simulink model "torque_control_180"  (R2021a)
settings: Solver=FixedStepAuto  StartTime=0.0  StopTime=1  FixedStep=1e-6  MaxStep=1e-6  RelTol=1e-3
values from neighbouring files (symbols this model uses):
  P = 8    [Arrow_86EMB3S98F_specs.m]    (also in M_2311P_specs.m)
undefined symbols (not defined in the file or in its folder): DiscIntNeverNeededParam, J, k1, k2, lambda_md, lls, rs, vdc
libraries: simulink x19, spsIGBTDiodeLib x6, spsSeriesRLCBranchLib x4, spsVoltageMeasurementLib x4, spsControlledCurrentSourceLib x3, spsGroundLib x2, spsControlledVoltageSourceLib x1, spspowerguiLib x1
settings Model: Creator=zlfen019.stu  LastModifiedBy=zlfen019.stu
settings DataIOCC: ReturnWorkspaceOutputs=off

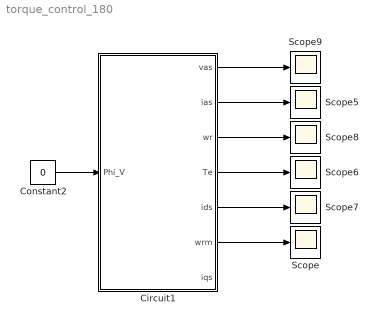
== system torque_control_180 ==
  Circuit1 : Subsystem
  Constant2 : Constant  Value=0
  Scope{,5..9} (6 alike) : Scope
  wires:
  Constant2/1 -> Circuit1/1(Phi_V)
  Circuit1/4(Te) -> Scope6/1
  Circuit1/5(ids) -> Scope7/1
  Circuit1/3(wr) -> Scope8/1
  Circuit1/2(ias) -> Scope5/1
  Circuit1/1(vas) -> Scope9/1
  Circuit1/6(wrm) -> Scope/1

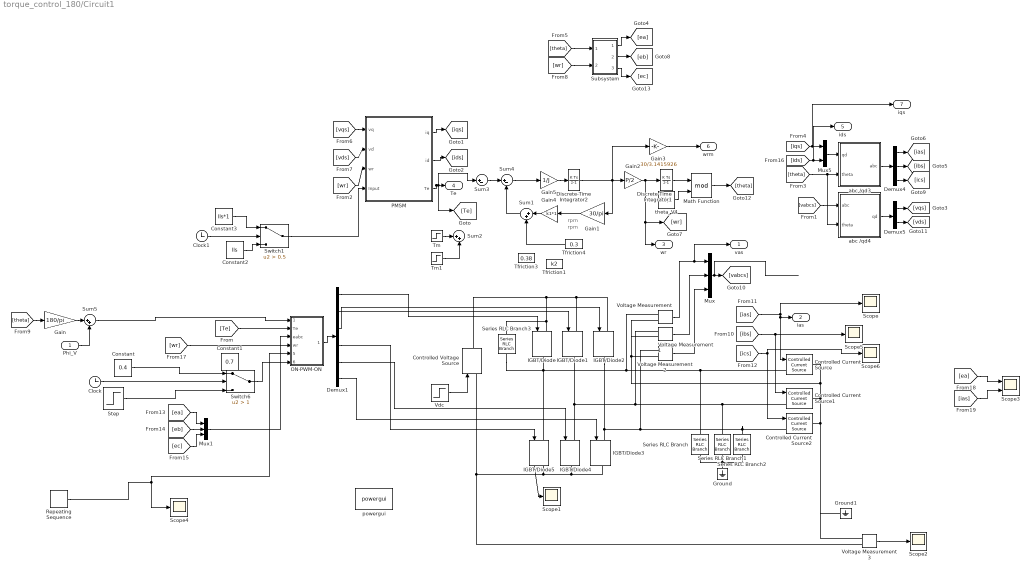
== system torque_control_180/Circuit1 ==
  note: rpm
  note: rpm
  Phi_V : Inport
  Clock : Clock
  Clock1 : Clock
  Constant : Constant  Value=0.4
  Constant1 : Constant  Value=0.7
  Constant2 : Constant  Value=lls
  Constant3 : Constant  Value=lls*1
  Controlled Current Source : spsControlledCurrentSourceLib/Controlled Current Source  Initialize=on  Source_Type=AC  Amplitude=0  Phase=0  Frequency=0  Measurements=None
  Controlled Current Source1 : spsControlledCurrentSourceLib/Controlled Current Source  Initialize=on  Source_Type=AC  Amplitude=0  Phase=0  Frequency=0  Measurements=None
  Controlled Current Source2 : spsControlledCurrentSourceLib/Controlled Current Source  Initialize=on  Source_Type=AC  Amplitude=0  Phase=0  Frequency=0  Measurements=None
  Controlled Voltage Source : spsControlledVoltageSourceLib/Controlled Voltage Source  Initialize=off  Source_Type=AC  Amplitude=0  Phase=0  Frequency=0  Measurements=None
  Demux1 : Demux  Outputs=6
  Demux4 : Demux  Outputs=3
  Demux5 : Demux  Outputs=2
  Discrete-Time Integrator1 : DiscreteIntegrator  SampleTime=-1  ICPrevOutput=DiscIntNeverNeededParam  ICPrevScaledInput=DiscIntNeverNeededParam
  Discrete-Time Integrator2 : DiscreteIntegrator  SampleTime=-1  ICPrevOutput=DiscIntNeverNeededParam  ICPrevScaledInput=DiscIntNeverNeededParam
  Gain : Gain  Gain=180/pi
  Gain1 : Gain  Gain=30/pi
  Gain2 : Gain  Gain=P/2
  Gain3 : Gain  Gain=30/3.1415926
  Gain4 : Gain  Gain=k1*1
  Gain5 : Gain  Gain=1/J
  Ground : spsGroundLib/Ground  LConnTagsString=a
  Ground1 : spsGroundLib/Ground  LConnTagsString=a
  IGBT/Diode{,1..4} (5 alike) : spsIGBTDiodeLib/IGBT//Diode  Ron=1e-3  Rs=inf  Cs=inf  Measurements=off
  IGBT/Diode5 : spsIGBTDiodeLib/IGBT//Diode  Ron=1e-3  Rs=inf  Cs=inf  Measurements=on
  Math Function : Math  Operator=mod  SignedPower=on  SaturateOnIntegerOverflow=on
  Mux : Mux  Inputs=3
  Mux1 : Mux  Inputs=3
  Mux5 : Mux  Inputs=2
  ON-PWM-ON : Subsystem  TreatAsAtomicUnit=on
  PMSM : Subsystem
  Repeating Sequence : simulink/Sources/Repeating Sequence  rep_seq_t=[0 0.25e-4 0.5e-4]  rep_seq_y=[0 1 0]
  Scope{,1..2,4..6} (6 alike) : Scope
  Scope3 : Scope  NumInputPorts=2
  Series RLC Branch{,1..3} (4 alike) : spsSeriesRLCBranchLib/Series RLC Branch  LConnTagsString=__new0  RConnTagsString=__new0  BranchType=R  Resistance=1e6  Inductance=1e-3  SetiL0=off  InitialCurrent=0  Capacitance=1e-6  Setx0=off  InitialVoltage=0  Measurements=None
  Step : Step  Time=0.85  Before=0.635  After=0.635  SampleTime=0
  Subsystem : Subsystem
  Sum1 : Sum  Inputs=|++
  Sum2 : Sum  Inputs=|++
  Sum3 : Sum  Inputs=|+-  AccumDataTypeStr=single  OutDataTypeStr=single
  Sum4 : Sum  Inputs=|+-  OutDataTypeStr=double
  Sum5 : Sum  Inputs=|++
  Switch1 : Switch  Criteria=u2 > Threshold  Threshold=0.5
  Switch6 : Switch  Criteria=u2 > Threshold  Threshold=1
  Tfriction1 : Constant  Value=k2
  Tfriction3 : Constant  Value=0.38
  Tfriction4 : Constant  Value=0.3
  Tm : Step  Time=0.15  Before=3  After=3  SampleTime=0
  Tm1 : Step  After=0.5  SampleTime=0
  "Vdc " : Step  Time=2  Before=vdc  After=vdc  SampleTime=0
  Voltage Measurement{,1..3} (4 alike) : spsVoltageMeasurementLib/Voltage Measurement  PhasorSimulation=off  OutputType=Complex  PSBequivalent=0
  abc /qd3 : Subsystem
  abc /qd4 : Subsystem
  powergui : spspowerguiLib/powergui  Priority=1  SimulationMode=Discrete  SampleTime=1e-6  frequency=60  Iterations=50  frequencyindice=0  Pbase=100e6  ErrMax=1e-4  UnitsV=kV  UnitsW=MW  buscounter=0  FunctionMessages=on  echomessages=off  EnableUseOfTLC=off  CurrentSourceSwitches=off  DisableSnubberDevices=off  DisableRonSwitches=on  DisableVfSwitches=on  DisplayEquations=off  AutomaticDiscreteSolvers=off  SolverType=Tustin/Backward Euler (TBE)  Interpol=off  ExternalGateDelay=off  methode=off  Ts=100  x0status=blocks  SPID=on  SwTol=0  HookPort=off  NonlinearTolerance=1e-4  nMaxIteration=100  ContinueOnMaxIteration=off  RestoreLinks=warning  ResistiveCurrentMeasurement=off  Frange=[0:2:500]  Ylog=off  Xlog=on  ShowGrid=off  save=off  variable=ZData  structure=ias  ZoomFFT=off  StartTime=0.1  cycles=230  DisplayStyle=1  fundamental=174  FreqAxis=on  MaxFrequency=2500  frequencyindicesteady=1  RmsSteady=1  display=off
  theta_V4 : Constant  Value=2*pi
  vas : Outport
  ias : Outport  Port=2
  wr : Outport  Port=3
  Te : Outport  Port=4
  ids : Outport  Port=5
  wrm : Outport  Port=6
  iqs : Outport  Port=7
  wires:
  Sum1/1 -> Sum4/2
  Repeating Sequence/1 -> ON-PWM-ON/5(Input), Scope4/1
  Gain4/1 -> Sum1/1
  Demux1/6 -> IGBT/Diode3/1
  Demux1/5 -> IGBT/Diode4/1
  Demux1/4 -> IGBT/Diode5/1
  Demux1/3 -> IGBT/Diode2/1
  Demux1/2 -> IGBT/Diode1/1
  Demux1/1 -> IGBT/Diode/1
  ON-PWM-ON/1(Output) -> Demux1/1
  Discrete-Time Integrator2/1 -> Gain3/1, Gain1/1, Gain2/1
  Sum4/1 -> Gain5/1
  Gain5/1 -> Discrete-Time Integrator2/1
  Gain2/1 -> Discrete-Time Integrator1/1, [wr], wr/1
  Math Function/1 -> [theta]
  Discrete-Time Integrator1/1 -> Math Function/1
  theta_V4/1 -> Math Function/2
  PMSM/3(Te) -> [Te], Sum3/1, Te/1
  Phi_V/1 -> Sum5/2
  Gain/1 -> Sum5/1
  [theta] -> Gain/1
  "Vdc "/1 -> Controlled Voltage Source/1
  [theta] -> abc /qd3/2(theta), abc /qd4/2(theta)
  Demux5/2 -> [vds]
  Demux5/1 -> [vqs]
  Demux4/3 -> [ics]
  Demux4/2 -> [ibs]
  Demux4/1 -> [ias]
  [ids] -> Mux5/2, ids/1
  [iqs] -> iqs/1, Mux5/1
  [vabcs] -> abc /qd4/1(abc)
  abc /qd3/1(abc) -> Demux4/1
  abc /qd4/1(qd) -> Demux5/1
  Mux5/1 -> abc /qd3/1(qd)
  PMSM/1(iq) -> [iqs]
  PMSM/2(id) -> [ids]
  [wr] -> PMSM/3(wr)
  [vds] -> PMSM/2(vd)
  [vqs] -> PMSM/1(vq)
  Mux/1 -> [vabcs]
  Voltage Measurement1/1 -> Mux/2
  Voltage Measurement2/1 -> Mux/3
  Voltage Measurement/1 -> Mux/1, vas/1
  [ics] -> Controlled Current Source2/1, Scope6/1
  [ibs] -> Controlled Current Source1/1, Scope5/1
  [ias] -> ias/1, Controlled Current Source/1, Scope/1
  IGBT/Diode5/1 -> Scope1/1
  Gain1/1 -> Gain4/1
  Tm1/1 -> Sum2/2
  Tm/1 -> Sum2/1
  Sum3/1 -> Sum4/1
  [Te] -> ON-PWM-ON/2(Te)
  [theta] -> Subsystem/1(Input)
  [wr] -> Subsystem/2(Input1)
  Subsystem/1(Output) -> [ea]
  Subsystem/2(Output1) -> [eb]
  Subsystem/3(Output2) -> [ec]
  Sum5/1 -> ON-PWM-ON/1(theta1)
  Mux1/1 -> ON-PWM-ON/3(eabc)
  [eb] -> Mux1/2
  [ea] -> Mux1/1
  [ec] -> Mux1/3
  [wr] -> ON-PWM-ON/4(wr)
  Voltage Measurement3/1 -> Scope2/1
  [ea] -> Scope3/1
  [ias] -> Scope3/2
  Gain3/1 -> wrm/1
  Clock/1 -> Switch6/2
  Constant/1 -> Switch6/1
  Step/1 -> Switch6/3
  Tfriction4/1 -> Sum1/2
  Switch6/1 -> ON-PWM-ON/6(Input1)
  Switch1/1 -> PMSM/4(Input)
  Constant2/1 -> Switch1/3
  Clock1/1 -> Switch1/2
  Constant3/1 -> Switch1/1
  connections:
  IGBT/Diode1/LConn1 -- IGBT/Diode2/LConn1 -- Controlled Voltage Source/RConn1 -- Series RLC Branch3/LConn1 -- IGBT/Diode/LConn1
  IGBT/Diode5/RConn1 -- Voltage Measurement3/LConn2 -- Controlled Voltage Source/LConn1 -- IGBT/Diode3/RConn1 -- IGBT/Diode4/RConn1
  Controlled Current Source2/LConn1 -- Series RLC Branch2/LConn1 -- Voltage Measurement2/LConn1 -- IGBT/Diode2/RConn1 -- IGBT/Diode3/LConn1
  Controlled Current Source1/LConn1 -- Series RLC Branch1/LConn1 -- Voltage Measurement1/LConn1 -- IGBT/Diode4/LConn1 -- IGBT/Diode1/RConn1
  Controlled Current Source/LConn1 -- Series RLC Branch/LConn1 -- Voltage Measurement/LConn1 -- Series RLC Branch3/RConn1 -- IGBT/Diode5/LConn1 -- IGBT/Diode/RConn1
  Ground/LConn1 -- Series RLC Branch2/RConn1 -- Series RLC Branch/RConn1 -- Series RLC Branch1/RConn1
  Controlled Current Source/RConn1 -- Voltage Measurement/LConn2 -- Voltage Measurement1/LConn2 -- Voltage Measurement2/LConn2 -- Voltage Measurement3/LConn1 -- Ground1/LConn1 -- Controlled Current Source2/RConn1 -- Controlled Current Source1/RConn1

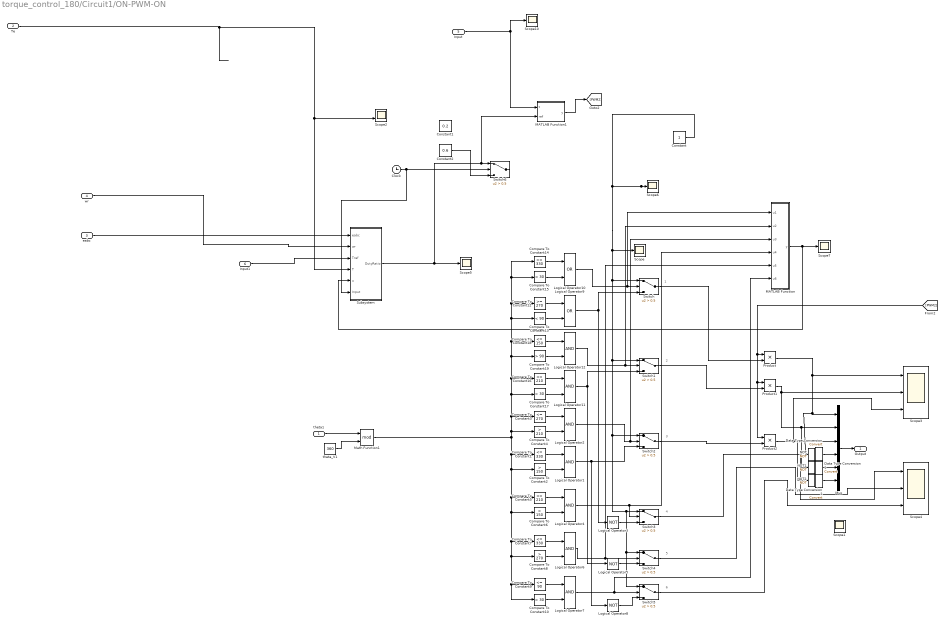
== system torque_control_180/Circuit1/ON-PWM-ON ==
  note: 6
  note: 4
  note: 3
  note: 2
  note: 1
  note: 5
  theta1 : Inport
  Te : Inport  Port=2
  eabc : Inport  Port=3
  wr : Inport  Port=4
  Input : Inport  Port=5
  Input1 : Inport  Port=6
  Clock : Clock
  Compare To Constant1 : simulink/Logic and Bit Operations/Compare To Constant  relop=<=  const=330  OutDataTypeStr=uint8
  Compare To Constant10 : simulink/Logic and Bit Operations/Compare To Constant  relop=>  const=30  OutDataTypeStr=uint8
  Compare To Constant12 : simulink/Logic and Bit Operations/Compare To Constant  relop=>=  const=270  OutDataTypeStr=uint8
  Compare To Constant13 : simulink/Logic and Bit Operations/Compare To Constant  relop=<  const=90  OutDataTypeStr=uint8
  Compare To Constant14 : simulink/Logic and Bit Operations/Compare To Constant  relop=>=  const=330  OutDataTypeStr=uint8
  Compare To Constant15 : simulink/Logic and Bit Operations/Compare To Constant  relop=<  const=30  OutDataTypeStr=uint8
  Compare To Constant16 : simulink/Logic and Bit Operations/Compare To Constant  relop=<=  const=210  OutDataTypeStr=uint8
  Compare To Constant17 : simulink/Logic and Bit Operations/Compare To Constant  relop=>  const=30  OutDataTypeStr=uint8
  Compare To Constant18 : simulink/Logic and Bit Operations/Compare To Constant  relop=<=  const=150  OutDataTypeStr=uint8
  Compare To Constant19 : simulink/Logic and Bit Operations/Compare To Constant  relop=>  const=90  OutDataTypeStr=uint8
  Compare To Constant2 : simulink/Logic and Bit Operations/Compare To Constant  relop=>  const=150  OutDataTypeStr=uint8
  Compare To Constant3 : simulink/Logic and Bit Operations/Compare To Constant  relop=<=  const=270  OutDataTypeStr=uint8
  Compare To Constant4 : simulink/Logic and Bit Operations/Compare To Constant  relop=>  const=210  OutDataTypeStr=uint8
  Compare To Constant5 : simulink/Logic and Bit Operations/Compare To Constant  relop=<=  const=210  OutDataTypeStr=uint8
  Compare To Constant6 : simulink/Logic and Bit Operations/Compare To Constant  relop=>  const=150  OutDataTypeStr=uint8
  Compare To Constant7 : simulink/Logic and Bit Operations/Compare To Constant  relop=<=  const=330  OutDataTypeStr=uint8
  Compare To Constant8 : simulink/Logic and Bit Operations/Compare To Constant  relop=>  const=270  OutDataTypeStr=uint8
  Compare To Constant9 : simulink/Logic and Bit Operations/Compare To Constant  relop=<=  const=90  OutDataTypeStr=uint8
  Constant : Constant
  Constant1 : Constant  Value=0.2
  Constant2 : Constant  Value=0.6
  Data Type Conversion : DataTypeConversion
  Data Type Conversion1 : DataTypeConversion
  Data Type Conversion2 : DataTypeConversion
  Logical Operator{1..2,4,6..7,11..12} (7 alike) : Logic  AllPortsSameDT=off  OutDataTypeStr=boolean
  Logical Operator10 : Logic  Operator=OR  AllPortsSameDT=off  OutDataTypeStr=boolean
  Logical Operator3 : Logic  Operator=NOT  AllPortsSameDT=off  OutDataTypeStr=boolean
  Logical Operator5 : Logic  Operator=NOT  AllPortsSameDT=off  OutDataTypeStr=boolean
  Logical Operator8 : Logic  Operator=NOT  AllPortsSameDT=off  OutDataTypeStr=boolean
  Logical Operator9 : Logic  Operator=OR  AllPortsSameDT=off  OutDataTypeStr=boolean
  MATLAB Function : MATLAB Function  TreatAsAtomicUnit=on
  MATLAB Function1 : MATLAB Function  TreatAsAtomicUnit=on
  Math Function1 : Math  Operator=mod  SignedPower=on  SaturateOnIntegerOverflow=on
  Mux : Mux  Inputs=6
  NOT : Logic  Operator=NOT  IconShape=distinctive  AllPortsSameDT=off  OutDataTypeStr=boolean
  NOT1 : Logic  Operator=NOT  IconShape=distinctive  AllPortsSameDT=off  OutDataTypeStr=boolean
  NOT2 : Logic  Operator=NOT  IconShape=distinctive  AllPortsSameDT=off  OutDataTypeStr=boolean
  Product : Product
  Product1 : Product
  Product2 : Product
  Scope{,1,5..7,10} (6 alike) : Scope
  Scope2 : Scope  NumInputPorts=2
  Scope3 : Scope  NumInputPorts=3
  Scope4 : Scope  NumInputPorts=3
  Subsystem : Subsystem  TreatAsAtomicUnit=on  SystemSampleTime=0.5e-4
  Switch{,1..6} (7 alike) : Switch  Criteria=u2 > Threshold  Threshold=0.5
  theta_V1 : Constant  Value=360
  Output : Outport
  wires:
  Constant/1 -> Scope6/1, Switch4/1, Switch5/1, Switch3/1, Switch2/1, Switch1/1, Switch/1, Scope/1
  Input/1 -> Scope10/1, MATLAB Function1/1(t)
  theta_V1/1 -> Math Function1/2
  theta1/1 -> Math Function1/1
  Compare To Constant12/1 -> Logical Operator9/1
  Compare To Constant13/1 -> Logical Operator9/2
  Logical Operator9/1 -> Logical Operator3/1, Switch/3
  Compare To Constant14/1 -> Logical Operator10/1
  Compare To Constant15/1 -> Logical Operator10/2
  Logical Operator10/1 -> MATLAB Function/1(u1), Switch/2
  Compare To Constant17/1 -> Logical Operator11/2
  Compare To Constant16/1 -> Logical Operator11/1
  Compare To Constant18/1 -> Logical Operator12/1
  Compare To Constant19/1 -> Logical Operator12/2
  Logical Operator12/1 -> MATLAB Function/2(u2), Switch1/2
  Logical Operator11/1 -> Switch1/3, Logical Operator5/1
  Logical Operator1/1 -> Logical Operator8/1, Switch2/3
  Logical Operator2/1 -> MATLAB Function/3(u3), Switch2/2
  Compare To Constant4/1 -> Logical Operator2/2
  Compare To Constant3/1 -> Logical Operator2/1
  Compare To Constant1/1 -> Logical Operator1/1
  Compare To Constant2/1 -> Logical Operator1/2
  Logical Operator3/1 -> Switch3/3
  Compare To Constant6/1 -> Logical Operator4/2
  Compare To Constant5/1 -> Logical Operator4/1
  Logical Operator4/1 -> MATLAB Function/4(u4), Switch3/2
  Logical Operator5/1 -> Switch4/3
  Compare To Constant7/1 -> Logical Operator6/1
  Compare To Constant8/1 -> Logical Operator6/2
  Logical Operator6/1 -> MATLAB Function/5(u5), Switch4/2
  Compare To Constant10/1 -> Logical Operator7/2
  Compare To Constant9/1 -> Logical Operator7/1
  Math Function1/1 -> Compare To Constant9/1, Compare To Constant10/1, Compare To Constant8/1, Compare To Constant7/1, Compare To Constant6/1, Compare To Constant5/1, Compare To Constant2/1, Compare To Constant1/1, Compare To Constant14/1, Compare To Constant15/1, Compare To Constant12/1, Compare To Constant13/1, Compare To Constant18/1, Compare To Constant19/1, Compare To Constant16/1, Compare To Constant17/1, Compare To Constant3/1, Compare To Constant4/1
  Logical Operator7/1 -> MATLAB Function/6(u6), Switch5/2
  Logical Operator8/1 -> Switch5/3
  Switch3/1 -> Scope4/1
  Switch4/1 -> Scope4/2
  Switch5/1 -> Scope4/3
  Mux/1 -> Output/1
  eabc/1 -> Subsystem/1(eabc)
  wr/1 -> Subsystem/2(wr)
  Te/1 -> Subsystem/4(T), Scope2/2
  MATLAB Function/1(y) -> Scope7/1, Subsystem/5(u)
  MATLAB Function1/1(y) -> [PWM2]
  Input1/1 -> Subsystem/3(Tref)
  Switch/1 -> Product/2
  [PWM2] -> Product2/1, Product1/1, Product/1
  Product/1 -> Scope3/1, NOT/1, Mux/1
  Switch1/1 -> Product1/2
  Product1/1 -> Scope3/2, NOT1/1, Mux/2
  Switch2/1 -> Product2/2
  Product2/1 -> Scope3/3, NOT2/1, Mux/3
  Clock/1 -> Subsystem/6(Input), Switch6/2
  Subsystem/1(DutyRatio) -> MATLAB Function1/2(ref), Switch6/1, Scope5/1
  Constant2/1 -> Switch6/3
  NOT/1 -> Data Type Conversion/1
  Data Type Conversion/1 -> Mux/4
  Data Type Conversion1/1 -> Mux/5
  NOT1/1 -> Data Type Conversion1/1
  NOT2/1 -> Data Type Conversion2/1
  Data Type Conversion2/1 -> Mux/6

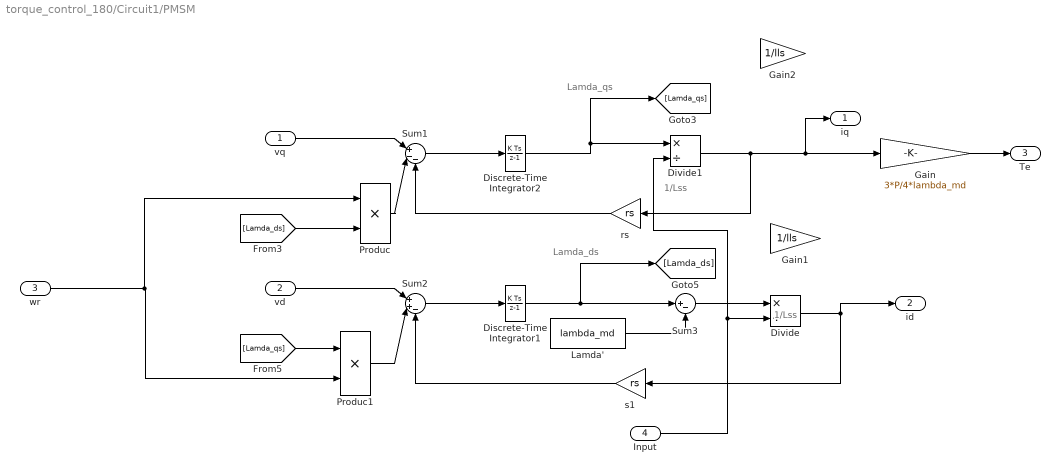
== system torque_control_180/Circuit1/PMSM ==
  note: Lamda_ds
  note: Lamda_qs
  note: 1/Lss
  note: 1/Lss
  vq : Inport
  vd : Inport  Port=2
  wr : Inport  Port=3
  Input : Inport  Port=4
  Discrete-Time Integrator1 : DiscreteIntegrator  SampleTime=-1  ICPrevOutput=DiscIntNeverNeededParam  ICPrevScaledInput=DiscIntNeverNeededParam
  Discrete-Time Integrator2 : DiscreteIntegrator  SampleTime=-1  ICPrevOutput=DiscIntNeverNeededParam  ICPrevScaledInput=DiscIntNeverNeededParam
  Divide : Product  Inputs=*/
  Divide1 : Product  Inputs=*/
  Gain : Gain  Gain=3*P/4*lambda_md
  Gain1 : Gain  Gain=1/lls
  Gain2 : Gain  Gain=1/lls
  Lamda' : Constant  Value=lambda_md
  Produc : Product  RndMeth=Zero
  Produc1 : Product  RndMeth=Zero
  Sum1 : Sum  Inputs=|+--
  Sum2 : Sum  Inputs=|++-
  Sum3 : Sum  Inputs=|+-
  rs : Gain  Gain=rs
  s1 : Gain  Gain=rs
  iq : Outport
  id : Outport  Port=2
  Te : Outport  Port=3
  wires:
  vd/1 -> Sum2/1
  vq/1 -> Sum1/1
  [Lamda_qs] -> Produc1/1
  [Lamda_ds] -> Produc/2
  wr/1 -> Produc1/2, Produc/1
  Lamda'/1 -> Sum3/2
  Sum3/1 -> Divide/1
  s1/1 -> Sum2/3
  Discrete-Time Integrator1/1 -> [Lamda_ds], Sum3/1
  Sum2/1 -> Discrete-Time Integrator1/1
  Produc1/1 -> Sum2/2
  Divide1/1 -> rs/1, Gain/1, iq/1
  rs/1 -> Sum1/3
  Discrete-Time Integrator2/1 -> Divide1/1, [Lamda_qs]
  Sum1/1 -> Discrete-Time Integrator2/1
  Produc/1 -> Sum1/2
  Gain/1 -> Te/1
  Divide/1 -> id/1, s1/1
  Input/1 -> Divide/2, Divide1/2

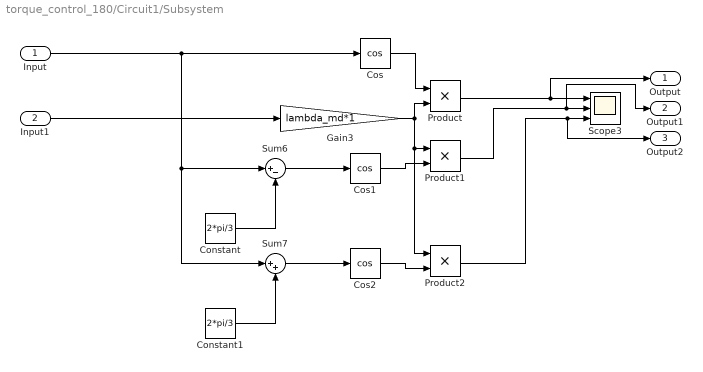
== system torque_control_180/Circuit1/Subsystem ==
  Input : Inport
  Input1 : Inport  Port=2
  Constant : Constant  Value=2*pi/3
  Constant1 : Constant  Value=2*pi/3
  Cos : Trigonometry  Operator=cos
  Cos1 : Trigonometry  Operator=cos
  Cos2 : Trigonometry  Operator=cos
  Gain3 : Gain  Gain=lambda_md*1
  Product : Product
  Product1 : Product
  Product2 : Product
  Scope3 : Scope  NumInputPorts=3
  Sum6 : Sum  Inputs=|+-  AccumDataTypeStr=single  OutDataTypeStr=single
  Sum7 : Sum  Inputs=|++  AccumDataTypeStr=single  OutDataTypeStr=single
  Output : Outport
  Output1 : Outport  Port=2
  Output2 : Outport  Port=3
  wires:
  Constant/1 -> Sum6/2
  Gain3/1 -> Product2/1, Product1/1, Product/2
  Cos2/1 -> Product2/2
  Cos/1 -> Product/1
  Cos1/1 -> Product1/2
  Product1/1 -> Output1/1, Scope3/2
  Product/1 -> Output/1, Scope3/1
  Sum7/1 -> Cos2/1
  Sum6/1 -> Cos1/1
  Product2/1 -> Output2/1, Scope3/3
  Constant1/1 -> Sum7/2
  Input/1 -> Cos/1, Sum7/1, Sum6/1
  Input1/1 -> Gain3/1

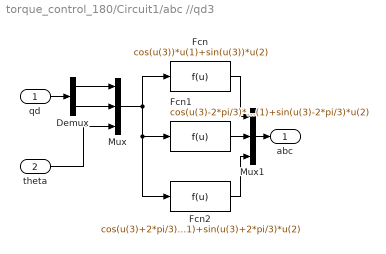
== system torque_control_180/Circuit1/abc //qd3 ==
  qd : Inport
  theta : Inport  Port=2
  Demux : Demux  Outputs=2
  Fcn : Fcn  Expr=cos(u(3))*u(1)+sin(u(3))*u(2)
  Fcn1 : Fcn  Expr=cos(u(3)-2*pi/3)*u(1)+sin(u(3)-2*pi/3)*u(2)
  Fcn2 : Fcn  Expr=cos(u(3)+2*pi/3)*u(1)+sin(u(3)+2*pi/3)*u(2)
  Mux : Mux  Inputs=3
  Mux1 : Mux  Inputs=3
  abc : Outport
  wires:
  Fcn2/1 -> Mux1/3
  Fcn/1 -> Mux1/1
  Mux1/1 -> abc/1
  Fcn1/1 -> Mux1/2
  qd/1 -> Demux/1
  Mux/1 -> Fcn/1, Fcn2/1, Fcn1/1
  Demux/1 -> Mux/1
  Demux/2 -> Mux/2
  theta/1 -> Mux/3

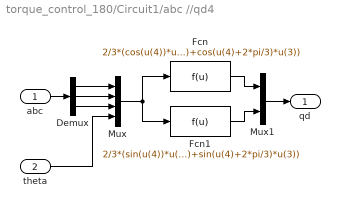
== system torque_control_180/Circuit1/abc //qd4 ==
  abc : Inport
  theta : Inport  Port=2
  Demux : Demux  Outputs=3
  Fcn : Fcn  Expr=2/3*(cos(u(4))*u(1)+cos(u(4)-2*pi/3)*u(2)+cos(u(4)+2*pi/3)*u(3))
  Fcn1 : Fcn  Expr=2/3*(sin(u(4))*u(1)+sin(u(4)-2*pi/3)*u(2)+sin(u(4)+2*pi/3)*u(3))
  Mux : Mux
  Mux1 : Mux  Inputs=2
  qd : Outport
  wires:
  Mux1/1 -> qd/1
  Fcn1/1 -> Mux1/2
  Fcn/1 -> Mux1/1
  Mux/1 -> Fcn1/1, Fcn/1
  theta/1 -> Mux/4
  Demux/3 -> Mux/3
  Demux/2 -> Mux/2
  Demux/1 -> Mux/1
  abc/1 -> Demux/1

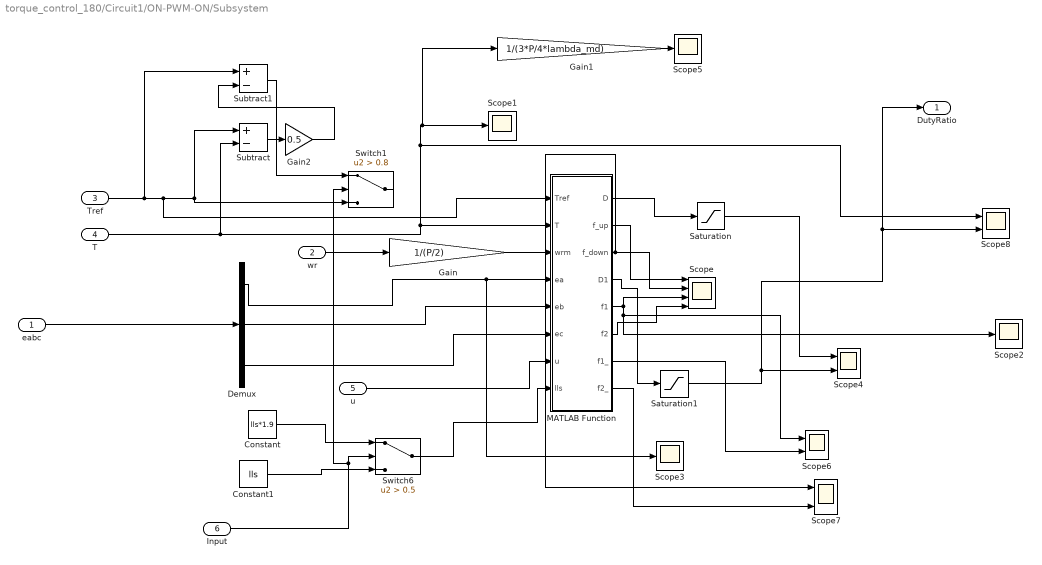
== system torque_control_180/Circuit1/ON-PWM-ON/Subsystem ==
  eabc : Inport
  wr : Inport  Port=2
  Tref : Inport  Port=3
  T : Inport  Port=4
  u : Inport  Port=5
  Input : Inport  Port=6
  Constant : Constant  Value=lls*1.9
  Constant1 : Constant  Value=lls
  Demux : Demux  Outputs=3
  Gain : Gain  Gain=1/(P/2)
  Gain1 : Gain  Gain=1/(3*P/4*lambda_md)
  Gain2 : Gain  Gain=0.5
  MATLAB Function : MATLAB Function  TreatAsAtomicUnit=on
  Saturation : Saturate  UpperLimit=1  LowerLimit=0
  Saturation1 : Saturate  UpperLimit=1  LowerLimit=0.1
  Scope : Scope  NumInputPorts=4
  Scope{1..3,5} (4 alike) : Scope
  Scope{4,6..8} (4 alike) : Scope  NumInputPorts=2
  Subtract : Sum  Inputs=+-
  Subtract1 : Sum  Inputs=+-
  Switch1 : Switch  Criteria=u2 > Threshold  Threshold=0.8
  Switch6 : Switch  Criteria=u2 > Threshold  Threshold=0.5
  DutyRatio : Outport
  wires:
  Gain/1 -> MATLAB Function/3(wrm)
  MATLAB Function/6(f2) -> Scope/4
  MATLAB Function/5(f1) -> Scope6/1, Scope2/1, Scope/3
  Saturation1/1 -> Scope8/2, DutyRatio/1, Scope4/2
  MATLAB Function/4(D1) -> Saturation1/1
  Saturation/1 -> Scope4/1
  eabc/1 -> Demux/1
  Demux/1 -> MATLAB Function/4(ea), Scope3/1
  Demux/2 -> MATLAB Function/5(eb)
  Demux/3 -> MATLAB Function/6(ec)
  Tref/1 -> Subtract1/1, MATLAB Function/1(Tref), Subtract/1, Switch1/3
  wr/1 -> Gain/1
  T/1 -> Subtract/2, Scope8/1, Gain1/1, Scope1/1, MATLAB Function/2(T)
  MATLAB Function/1(D) -> Saturation/1
  u/1 -> MATLAB Function/7(u)
  MATLAB Function/2(f_up) -> Scope/1
  MATLAB Function/7(f1_) -> Scope6/2
  MATLAB Function/8(f2_) -> Scope7/2
  MATLAB Function/3(f_down) -> Scope7/1, Scope/2
  Gain1/1 -> Scope5/1
  Input/1 -> Switch1/2, Switch6/2
  Constant/1 -> Switch6/1
  Constant1/1 -> Switch6/3
  Switch6/1 -> MATLAB Function/8(lls)
  Subtract/1 -> Gain2/1
  Gain2/1 -> Subtract1/2
  Subtract1/1 -> Switch1/1

== matlab function torque_control_180/Circuit1/ON-PWM-ON/MATLAB Function ==
  data: u1 input; y output; u2 input; u3 input; u4 input; u5 input; u6 input
function y = fcn(u1,u2,u3,u4,u5,u6)

if((u1==1)||(u4==1))
    y = 1;
elseif((u2==1)||(u5==1))
    y=2;
elseif((u3==1)||(u6==1))
    y=3;
else
    y=0;
end

== matlab function torque_control_180/Circuit1/ON-PWM-ON/Subsystem/MATLAB Function ==
  data: Tref input; D output; T input; wrm input; ea input; eb input; ec input; u input; f_up output; f_down output; D1 output; f1 output; f2 output; vdc parameter; rs parameter; f1_ output; f2_ output; lls input
function [D,f_up,f_down,D1,f1,f2,f1_,f2_] = fcn(Tref,T,wrm,ea,eb,ec, u, vdc, rs, lls)


if (u == 1)
D = (-Tref+T)*wrm*lls/(0.5e-4)/vdc/abs(ea)+1-(ea^2+eb^2+ec^2)/vdc/abs(ea);
f_up = ((abs(ea)*vdc-(ea^2+eb^2+ec^2))/wrm/lls)%-rs/lls*T%;
f_down = -(ea^2+eb^2+ec^2)/wrm/lls%-rs/lls*T%;

elseif (u == 2)
D = (-Tref+T)*wrm*lls/(0.5e-4)/vdc/abs(eb)+1-(ea^2+eb^2+ec^2)/vdc/abs(eb);
f_up = (abs(eb)*vdc-(ea^2+eb^2+ec^2))/wrm/lls%-rs/lls*T%;
f_down = -(ea^2+eb^2+ec^2)/wrm/lls%-rs/lls*T%;

else
D = (-Tref+T)*wrm*lls/(0.5e-4)/vdc/abs(ec)+1-(ea^2+eb^2+ec^2)/vdc/abs(ec);
f_up = (abs(ec)*vdc-(ea^2+eb^2+ec^2))/wrm/lls%-rs/lls*T%;
f_down = -(ea^2+eb^2+ec^2)/wrm/lls%-rs/lls*T%;

end
f2 = f_down;
f1 = abs(f_up);
%D1 = 0;
f1_=(2*vdc*0.037*0.933-3*wrm*2*0.037^2)/lls %-rs/lls*T%;
f2_= -3*wrm*2*0.037^2/lls%-rs/lls*T%;

D1 = 1-(Tref - T - (0.5e-4)*f1)/(f2 - f1)/0.5e-4;

== matlab function torque_control_180/Circuit1/ON-PWM-ON/MATLAB Function1 ==
  data: t input; y output; ref input
function y = fcn(t,ref)

if(t >= ref)
    y = 0;
else
    y = 1;
end
